simulink model "internal_model_control101"  (R2023b)
settings: Solver=VariableStepAuto  StartTime=0.0  StopTime=60  RelTol=1e-3
undefined symbols (not defined in the file or in its folder): deadtime, deadtimem
libraries: cstblocks x3
settings Model: Creator=barsr  LastModifiedBy=barsr

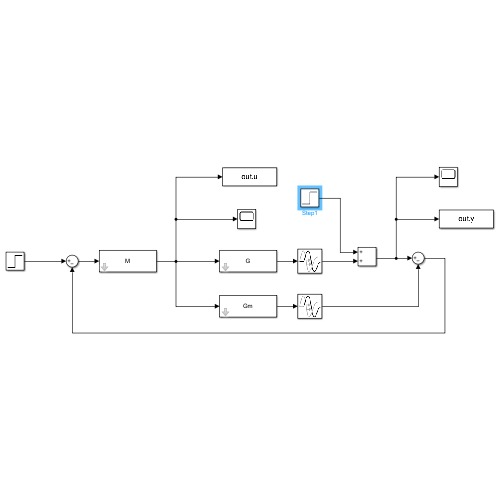
[thumbnail: Simulink's stored preview of the top-level diagram]
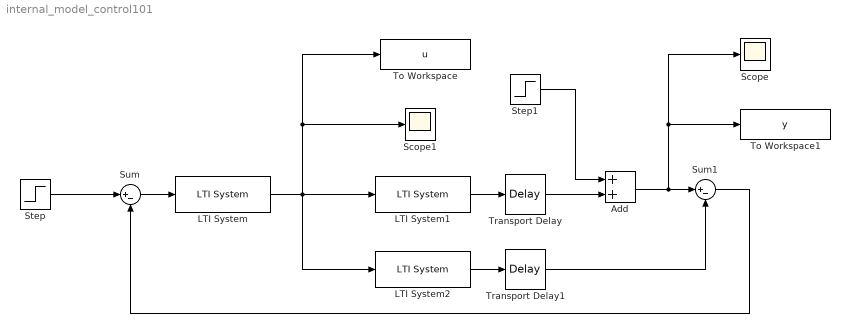
== system internal_model_control101 ==
  Add : Sum
  LTI System : cstblocks/LTI System  sys=M  IC=[]  PadeOrder=0
  LTI System1 : cstblocks/LTI System  sys=G  IC=[]  PadeOrder=0
  LTI System2 : cstblocks/LTI System  sys=Gm  IC=[]  PadeOrder=0
  Scope : Scope
  Scope1 : Scope
  Step : Step  Time=0  SampleTime=0
  Step1 : Step  Time=30  After=0.2  SampleTime=0
  Sum : Sum  Inputs=|+-
  Sum1 : Sum  Inputs=|+-
  To Workspace : ToWorkspace  VariableName=u  SaveFormat=Structure With Time  SampleTime=-1
  To Workspace1 : ToWorkspace  VariableName=y  SaveFormat=Structure With Time  SampleTime=-1
  Transport Delay : TransportDelay  DelayTime=deadtime
  Transport Delay1 : TransportDelay  DelayTime=deadtimem
  wires:
  Sum/1 -> LTI System/1
  LTI System1/1 -> Transport Delay/1
  LTI System/1 -> LTI System2/1, To Workspace/1, Scope1/1, LTI System1/1
  LTI System2/1 -> Transport Delay1/1
  Transport Delay1/1 -> Sum1/2
  Transport Delay/1 -> Add/2
  Step1/1 -> Add/1
  Add/1 -> Scope/1, To Workspace1/1, Sum1/1
  Sum1/1 -> Sum/2
  Step/1 -> Sum/1
